simulink model "p5p5f_d"  (Simulink 9.0)
settings: Solver=ode45  StartTime=0.0  StopTime=simtime  RelTol=1e-3  EnableMultiTasking=on
values from neighbouring files (symbols this model uses):
  K_bias = [0 0 0 0 1]    [Untitled_boi.m]    (also in p5p5c_init.m; p5p5d_init.m; p5p5e_init.m; p5p5f_d_init.m)
  K_psi = [0 0 1 0 0]    [Untitled_boi.m]    (also in p5p5c_init.m; p5p5d_init.m; p5p5e_init.m; p5p5f_d_init.m)
  ref = 30    [Untitled_boi.m]    (also in p5p5c_init.m; p5p5d_init.m; p5p5e_init.m; p5p5f_d_init.m)
  Ts = 0.10    (= 0.1)    [Untitled_boi.m]    (also in p5p5a_init.m; p5p5c_init.m; p5p5d_init.m; p5p5e_init.m)
libraries: simulink x2, cstblocks x1
settings Model: Creator=markh  LastModifiedBy=bruker
settings DataIOCC: LimitDataPoints=on  SignalLoggingSaveFormat=ModelDataLogs  SignalLoggingName=sigsOut
settings OptimizationCC: InitFltsAndDblsToZero=on
settings DebuggingCC: SaveWithParameterizedLinksMsg=none  SignalResolutionControl=TryResolveAllWithWarning  MultiTaskDSMMsg=warning  MultiTaskCondExecSysMsg=none  FcnCallInpInsideContextMsg=warning  StateNameClashWarn=warning
settings HardwareCC: TargetBitPerPointer=64  TargetBitPerSizeT=64  TargetBitPerPtrDiffT=64  TargetLongLongMode=on  TargetIntDivRoundTo=Zero  TargetEndianess=LittleEndian  TargetWordSize=64  TargetHWDeviceType=MATLAB Host  ProdEqTarget=off
settings GRTTargetCC: TargetFcnLib=ansi_tfl_tmw.mat  GeneratePreprocessorConditionals=Disable all  CombineOutputUpdateFcns=off  GRTInterface=on

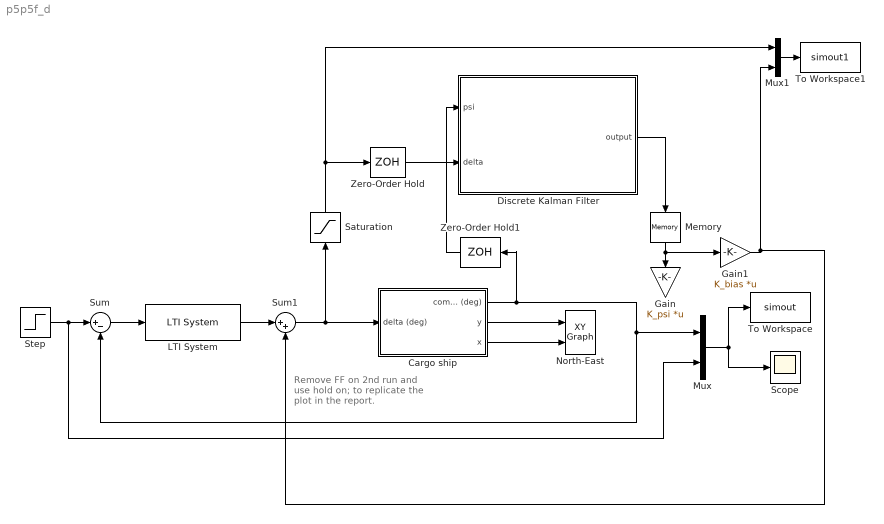
== system p5p5f_d ==
  note: Remove FF on 2nd run
      | and use hold on; to replicate
      | the plot in the report.
  Cargo ship : Subsystem  mask(Simple shipmodel for a cargo ship){noise=on, current=on, logic=off}
      mask prompts: noise "measurement noise"; logic "waves"
      mask help:
      | Measurement noise:
      | 	checked = noise on
      | 	unchecked = noise off
      |
      | Current:
      | 	checked = current on
      | 	unchecked = current off
      |
      | Waves:
      | 	checked = waves on
      | 	unchecked = waves off
      |
      | Author: Jørgen Spjøtvold, 9/10-2003
      | TTK 4115 Linear system theory.
      | Modified by Jostein Bakkeheim 26/10-2006
  Discrete Kalman Filter : MATLAB Function  TreatAsAtomicUnit=on
  Gain : Gain  Gain=K_psi  Multiplication=Matrix(K*u)
  Gain1 : Gain  Gain=K_bias  Multiplication=Matrix(K*u)
  LTI System : cstblocks/LTI System  sys=reg_sys  IC=[]
  Memory : Memory
  Mux : Mux  Inputs=2
  Mux1 : Mux  Inputs=2
  North-East : simulink/Sinks/XY Graph  xmin=-5000  xmax=5000  ymin=-5000  ymax=5000  st=-1
  Saturation : Saturate  UpperLimit=45  LowerLimit=-45
  Scope : Scope
  Step : Step  Time=0  After=ref  SampleTime=0
  Sum : Sum  Inputs=|+-
  Sum1 : Sum  Inputs=|++
  To Workspace : ToWorkspace  VariableName=simout  SaveFormat=Timeseries  SampleTime=-1
  To Workspace1 : ToWorkspace  VariableName=simout1  SaveFormat=Timeseries  SampleTime=-1
  Zero-Order Hold : ZeroOrderHold  SampleTime=Ts
  Zero-Order Hold1 : ZeroOrderHold  SampleTime=Ts
  wires:
  Cargo ship/3(x) -> North-East/2
  Cargo ship/2(y) -> North-East/1
  Step/1 -> Sum/1, Mux/2
  Sum/1 -> LTI System/1
  Mux/1 -> To Workspace/1, Scope/1
  Saturation/1 -> Mux1/1, Zero-Order Hold/1
  Memory/1 -> Gain1/1, Gain/1
  Zero-Order Hold/1 -> Discrete Kalman Filter/2(delta)
  Zero-Order Hold1/1 -> Discrete Kalman Filter/1(psi)
  Mux1/1 -> To Workspace1/1
  Discrete Kalman Filter/1(output) -> Memory/1
  Cargo ship/1(compass (deg)) -> Zero-Order Hold1/1, Mux/1, Sum/2
  LTI System/1 -> Sum1/1
  Sum1/1 -> Saturation/1, Cargo ship/1(delta (deg))
  Gain1/1 -> Sum1/2, Mux1/2

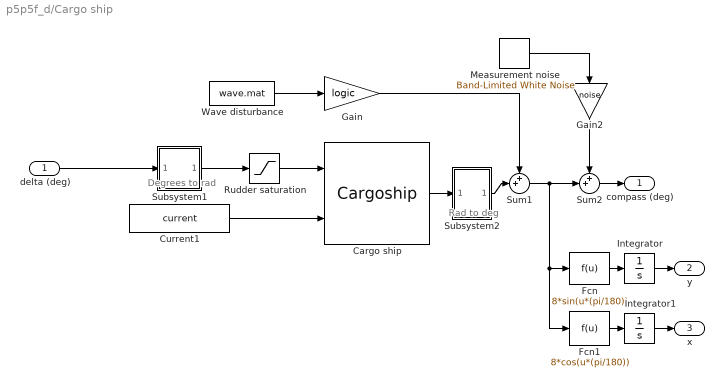
== system p5p5f_d/Cargo ship ==
  note: Degrees to rad
  note: Rad to deg
  delta (deg) : Inport
  Cargo ship : S-Function  FunctionName=Cargoship  SFunctionDeploymentMode=off  EnableBusSupport=off  mask(Cargo ship){}
      mask help:
      | S-function which simulates a cargo ship.
      |
      | Author: Jørgen Spjøtvold
      | 20.10-2003
      | Modified by Jostein Bakkeheim 27.10.2006
  Current1 : Constant  Value=current
  Fcn : Fcn  Expr=8*sin(u*(pi/180))
  Fcn1 : Fcn  Expr=8*cos(u*(pi/180))
  Gain : Gain  Gain=logic  SaturateOnIntegerOverflow=on  OutDataTypeStr=Inherit: Same as input  ParamDataTypeStr=Inherit: Same as input
  Gain2 : Gain  Gain=noise  SaturateOnIntegerOverflow=on  OutDataTypeStr=Inherit: Same as input  ParamDataTypeStr=Inherit: Same as input
  Integrator : Integrator
  Integrator1 : Integrator
  Measurement noise : simulink/Sources/Band-Limited White Noise  Cov=[0.001]  Ts=.5  seed=[23341]
  Rudder saturation : Saturate  UpperLimit=45*(pi/180)  LowerLimit=-45*(pi/180)
  Subsystem1 : Subsystem  mask(degrees to radians){}
      mask help: Converts degrees to radians
      mask Display: fprintf('D2R');
  Subsystem2 : Subsystem  mask(radians to degrees){}
      mask help: Converts radians to degrees
      mask Display: fprintf('R2D');
  Sum1 : Sum  Inputs=++|  SaturateOnIntegerOverflow=on
  Sum2 : Sum  Inputs=++|  SaturateOnIntegerOverflow=on
  Wave disturbance : FromFile  FileName=wave.mat  SampleTime=0
  compass (deg) : Outport
  y : Outport  Port=2
  x : Outport  Port=3
  wires:
  delta (deg)/1 -> Subsystem1/1(In1)
  Fcn/1 -> Integrator/1
  Integrator/1 -> y/1
  Fcn1/1 -> Integrator1/1
  Integrator1/1 -> x/1
  Wave disturbance/1 -> Gain/1
  Subsystem2/1(Out1) -> Sum1/2
  Gain/1 -> Sum1/1
  Sum1/1 -> Fcn/1, Fcn1/1, Sum2/2
  Cargo ship/1 -> Subsystem2/1(In1)
  Subsystem1/1(Out1) -> Rudder saturation/1
  Rudder saturation/1 -> Cargo ship/1
  Sum2/1 -> compass (deg)/1
  Measurement noise/1 -> Gain2/1
  Gain2/1 -> Sum2/1
  Current1/1 -> Cargo ship/2

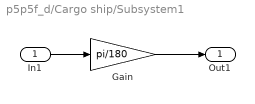
== system p5p5f_d/Cargo ship/Subsystem1 ==
  In1 : Inport
  Gain : Gain  Gain=pi/180  SaturateOnIntegerOverflow=on  OutDataTypeStr=Inherit: Same as input  ParamDataTypeStr=Inherit: Same as input
  Out1 : Outport
  wires:
  Gain/1 -> Out1/1
  In1/1 -> Gain/1

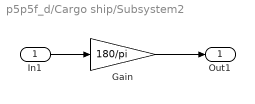
== system p5p5f_d/Cargo ship/Subsystem2 ==
  In1 : Inport
  Gain : Gain  Gain=180/pi  SaturateOnIntegerOverflow=on  OutDataTypeStr=Inherit: Same as input  ParamDataTypeStr=Inherit: Same as input
  Out1 : Outport
  wires:
  Gain/1 -> Out1/1
  In1/1 -> Gain/1

== matlab function Discrete Kalman Filter ==
  settings: updateMethod=DISCRETE  sampleTime=Ts
  data: psi input double; output output double size=5; delta input double; disc_struct parameter double
%function y = fcn(u)

%y = u;

% Discrete Kalman filter function
function output = DiscreteKalmanFilter(psi, delta, disc_struct)
 
    % system:
    % x_dot = A x + B u + G w
    % y = C x + v
 
    % static variables to update, including initialization flag
    persistent init_flag P_pri P x_est_pri x_est
    
    % from discretized model
    A_d = disc_struct.A_d;
    B_d = disc_struct.B_d;
    C_d = disc_struct.C_d;
    D_d = disc_struct.D_d;
    E_d = disc_struct.E_d;
    Q_d = disc_struct.Q_d;
    R_d = disc_struct.R_d;
   
    I = eye(5);
   
    % Initialization
    if (isempty(init_flag))
        init_flag = 1;
        x_est_pri = [0;
            0;
            0;
            0;
            0];
        
        P_pri = [1 0 0 0 0;
                    0 0.013 0 0 0;
                    0 0 (pi^(2)) 0 0;
                    0 0 0 1 0;
                    0 0 0 0 2.5*10^(-3)];
               
        %P_pri = P_pri_0;
        %x_est_pri = x_est_pri_0;
    end
   
    % computing Kalman gain
    K = P_pri * C_d.' * inv((C_d * P_pri * C_d.' + R_d));
   
    % update (a posteriori estimate) with blending factor/kalman gain
    x_est = x_est_pri + K * (psi - C_d * x_est_pri);
   
    % update error covariance matrix
    P = (I - K * C_d) * P_pri * (I - K * C_d).' + K * R_d * K.';
   
    % projecting ahead to next iteration
    x_est_pri = A_d * x_est + B_d * delta;
    P_pri = A_d * P * A_d.' + Q_d; % Q_d
   
    % return the a posteriori state estimate (extract psi and delta)
    output = x_est;
end
